simulink model "heat25830_staliro_02"  (R2021b)
settings: Solver=FixedStepAuto  StartTime=0  StopTime=50  FixedStep=0.05  RelTol=1e-5  AbsTol=1e-5  EnableMultiTasking=on
undefined symbols (not defined in the file or in its folder): Amat, bvec, cvec, dif, get, h, rooms, xinit
settings Model: Creator=gfaineko  LastModifiedBy=yangy
settings SolverCC: AutoScaleAbsTol=off  AlgebraicLoopSolver=TrustRegion
settings DataIOCC: ExternalInput=aoe_tsinghua_mhi_data  LoadExternalInput=on  SaveFormat=Array  SignalLoggingSaveFormat=ModelDataLogs  SaveOutput=off  SignalLogging=off  DSMLogging=off  SaveTime=off  ReturnWorkspaceOutputs=off  SignalLoggingName=sigsOut
settings OptimizationCC: ExpressionDepthLimit=2147483647  LifeSpan=inf
settings DebuggingCC: SaveWithParameterizedLinksMsg=none  UnderspecifiedInitializationDetection=Classic  MergeDetectMultiDrivingBlocksExec=none  SignalResolutionControl=TryResolveAllWithWarning  MultiTaskDSMMsg=warning  MultiTaskCondExecSysMsg=none  FcnCallInpInsideContextMsg=warning  StateNameClashWarn=warning  InitInArrayFormatMsg=none  SFUnexpectedBacktrackingDiag=warning  SFNoUnconditionalDefaultTransitionDiag=warning  SFExecutionAtInitializationDiag=none  SFMachineParentedDataDiag=warning  ArithmeticOperatorsInVariantConditions=warning
settings HardwareCC: ProdBitPerPointer=32  ProdBitPerSizeT=32  ProdBitPerPtrDiffT=32  ProdLargestAtomicFloat=None  ProdIntDivRoundTo=Undefined  ProdEndianess=Unspecified  ProdWordSize=32  ProdHWDeviceType=32-bit Generic  TargetUnknown=on
settings ModelReferenceCC: PropagateSignalLabelsOutOfModel=off
settings SFSimCC: SimUseLocalCustomCode=off  SimParseCustomCode=off  CustomCodeUndefinedFunction=UseInterfaceOnly
settings RTWCC: RTWUseLocalCustomCode=off
settings CodeAppCC: StateflowObjectComments=on
settings GRTTargetCC: TargetLangStandard=C89/C90 (ANSI)  CombineOutputUpdateFcns=off  GRTInterface=on
settings ConfigComp: CovMetricSettings=dw  CovSaveCumulativeToWorkspaceVar=on  CovSaveSingleToWorkspaceVar=on  CovExternalEMLEnable=off

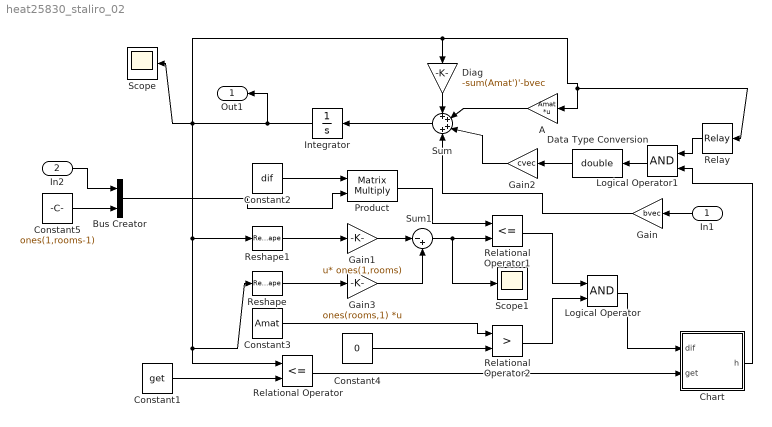
== system heat25830_staliro_02 ==
  In1 : Inport
  In2 : Inport  Port=2
  A : Gain  Gain=Amat  Multiplication=Matrix(K*u)  SaturateOnIntegerOverflow=on  OutDataTypeStr=Inherit: Same as input  ParamDataTypeStr=Inherit: Same as input
  Bus Creator : BusCreator  Inputs=2
  Chart : Stateflow chart  TreatAsAtomicUnit=on
  Constant1 : Constant  Value=get
  Constant2 : Constant  Value=dif
  Constant3 : Constant  Value=Amat  VectorParams1D=off
  Constant4 : Constant  Value=0
  Constant5 : Constant  Value=ones(1,rooms-1)  VectorParams1D=off
  Data Type Conversion : DataTypeConversion  OutDataTypeStr=double  SaturateOnIntegerOverflow=on  RndMeth=Zero
  Diag : Gain  Gain=-sum(Amat')'-bvec  SaturateOnIntegerOverflow=on  OutDataTypeStr=Inherit: Same as input  ParamDataTypeStr=Inherit: Same as input
  Gain : Gain  Gain=bvec  SaturateOnIntegerOverflow=on  OutDataTypeStr=Inherit: Same as input  ParamDataTypeStr=Inherit: Same as input
  Gain1 : Gain  Gain=ones(1,rooms)  Multiplication=Matrix(u*K)  SaturateOnIntegerOverflow=on  OutDataTypeStr=Inherit: Same as input  ParamDataTypeStr=Inherit: Same as input
  Gain2 : Gain  Gain=cvec  SaturateOnIntegerOverflow=on  OutDataTypeStr=Inherit: Same as input  ParamDataTypeStr=Inherit: Same as input
  Gain3 : Gain  Gain=ones(rooms,1)  Multiplication=Matrix(K*u)  SaturateOnIntegerOverflow=on  OutDataTypeStr=Inherit: Same as input  ParamDataTypeStr=Inherit: Same as input
  Integrator : Integrator  InitialCondition=xinit
  Logical Operator : Logic  AllPortsSameDT=off
  Logical Operator1 : Logic  AllPortsSameDT=off
  Product : Product  Multiplication=Matrix(*)  RndMeth=Zero
  Relational Operator : RelationalOperator  Operator=<=  OutDataTypeStr=boolean  RndMeth=Nearest
  Relational Operator1 : RelationalOperator  Operator=<=  OutDataTypeStr=boolean  RndMeth=Nearest
  Relational Operator2 : RelationalOperator  Operator=>  OutDataTypeStr=boolean  RndMeth=Nearest
  Relay : Relay  OnSwitchValue=off  OffSwitchValue=on  OnOutputValue=0  OffOutputValue=1
  Reshape : Reshape  OutputDimensionality=Row vector (2-D)
  Reshape1 : Reshape  OutputDimensionality=Column vector (2-D)
  Scope : Scope
  Scope1 : Scope
  Sum : Sum  Inputs=++++  SaturateOnIntegerOverflow=on
  Sum1 : Sum  Inputs=|-+  SaturateOnIntegerOverflow=on
  Out1 : Outport  VectorParamsAs1DForOutWhenUnconnected=off
  wires:
  Sum/1 -> Integrator/1
  Integrator/1 -> Scope/1, Relational Operator/1, Reshape/1, Reshape1/1, Diag/1, Relay/1, A/1, Out1/1
  Diag/1 -> Sum/1
  Relay/1 -> Logical Operator1/1
  Gain/1 -> Sum/4
  In1/1 -> Gain/1
  Relational Operator/1 -> Chart/2(get)
  Constant1/1 -> Relational Operator/2
  Reshape1/1 -> Gain1/1
  Reshape/1 -> Gain3/1
  Gain1/1 -> Sum1/1
  Gain3/1 -> Sum1/2
  Sum1/1 -> Scope1/1, Relational Operator1/2
  Product/1 -> Relational Operator1/1
  Relational Operator1/1 -> Logical Operator/1
  Constant3/1 -> Relational Operator2/1
  Constant4/1 -> Relational Operator2/2
  Relational Operator2/1 -> Logical Operator/2
  Logical Operator/1 -> Chart/1(dif)
  Logical Operator1/1 -> Data Type Conversion/1
  Data Type Conversion/1 -> Gain2/1
  Chart/1(h) -> Logical Operator1/2
  A/1 -> Sum/2
  Gain2/1 -> Sum/3
  Constant5/1 -> Bus Creator/2
  In2/1 -> Bus Creator/1
  Constant2/1 -> Product/1
  Bus Creator/1 -> Product/2

== stateflow chart heat25830_staliro_02/Chart ==
  state main [parallel]
    settings: executionOrder=1
    (junction 27) -> (junction 22) [order 1] : [id2<rooms]
    (junction 22) -> (junction 23)
    (junction 20) -> (junction 25) [order 1] : [id1<rooms]
    (junction 25) -> (junction 32)
    (junction 32) -> (junction 27) [order 1] : [get[id1]&!h[id1]]
    (junction 23) -> (junction 31) [order 1] : [dif[id1][id2]&h[id2]]
    (junction 29) -> (junction 27)
    (junction 27) -> (junction 21) [order 2] : {id2=0;}
    (junction 32) -> (junction 30) [order 2]
    (junction 23) -> (junction 29) [order 2] : {id2++;}
    (junction 31) -> (junction 28) : {h[id1]=1;h[id2]=0;}
    main -> (junction 20) : {id1=0;id2=0;}
    (junction 24) -> (junction 20)
    (junction 20) -> (junction 26) [order 2]
    (junction 21) -> (junction 30)
    (junction 30) -> (junction 24) : {id1++;}
    (junction 28) -> (junction 26)
    (junction 26) -> main
  data: id1 local int16; id2 local int16; rooms parameter double; dif input boolean size=10,10; get input boolean size=10; h output double size=10 =h
